simulink model "DOF4_model"  (R2023a)
settings: Solver=VariableStepAuto  StartTime=0.0  StopTime=10.0  RelTol=1e-3
values from neighbouring files (symbols this model uses):
  a = 1.8    [DOF_4_parameters.m]    (also in formulacar_params.mat; longitudinal_coefficients.m; roadcar_params.mat = 1.1)
  b = 1.7    [DOF_4_parameters.m]    (also in formulacar_params.mat; longitudinal_coefficients.m; roadcar_params.mat)
  c_damperF = 1580    [DOF_4_parameters.m]
  c_damperR = 1650    [DOF_4_parameters.m]
  F0F = m_s * (b / L) * g    (= 3740.41285714)    [DOF_4_parameters.m]
  F0R = m_s * (a / L) * g    (= 3960.43714286)    [DOF_4_parameters.m]
  g = 9.81    [DOF_4_parameters.m]    (also in formulacar_params.mat; longitudinal_coefficients.m; quarter_car_model_parameters.m; roadcar_params.mat)
  I = 1350    [DOF_4_parameters.m]    (also in formulacar_params.mat = 1500; roadcar_params.mat = 3500)
  k_springF = 37000    [DOF_4_parameters.m]
  k_springR = 47000    [DOF_4_parameters.m]
  k_tyreF = 400000    [DOF_4_parameters.m]
  k_tyreR = k_tyreF    (= 400000)    [DOF_4_parameters.m]
  m_s = 785    [DOF_4_parameters.m]    (also in quarter_car_model_parameters.m = 400)
  m_usF = 30    [DOF_4_parameters.m]
  m_usR = 35    [DOF_4_parameters.m]
  z0_tyreF = (m_s*b/L + m_usF) * g / k_tyreF    (= 0.0100867821429)    [DOF_4_parameters.m]
  z0_tyreR = (m_s*a/L + m_usF) * g / k_tyreR    (= 0.0106368428571)    [DOF_4_parameters.m]
  z_r_type = 1    [quarter_car_model_parameters.m]
libraries: simulink x1
settings Model: Creator=Cassio de Freitas  LastModifiedBy=Cassio de Freitas

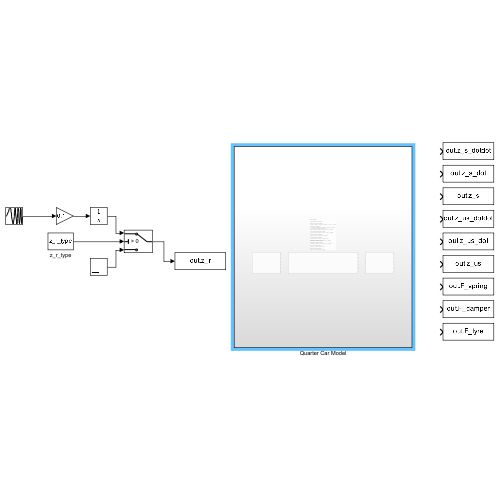
[thumbnail: Simulink's stored preview of the top-level diagram]
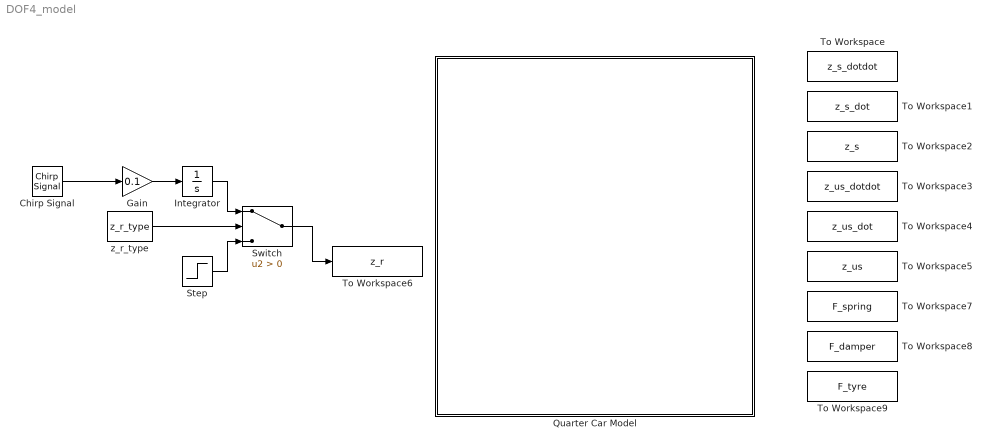
== system DOF4_model ==
  Chirp Signal : simulink/Sources/Chirp Signal  f1=0.1  T=100  f2=50
  Gain : Gain  Gain=0.1
  Integrator : Integrator
  Quarter Car Model : Subsystem
  Step : Step  After=0.1  SampleTime=1e-3
  Switch : Switch  Criteria=u2 > Threshold  SaturateOnIntegerOverflow=off  InputSameDT=off
  To Workspace : ToWorkspace  VariableName=z_s_dotdot  SaveFormat=Timeseries  SampleTime=-1
  To Workspace1 : ToWorkspace  VariableName=z_s_dot  SaveFormat=Timeseries  SampleTime=-1
  To Workspace2 : ToWorkspace  VariableName=z_s  SaveFormat=Timeseries  SampleTime=-1
  To Workspace3 : ToWorkspace  VariableName=z_us_dotdot  SaveFormat=Timeseries  SampleTime=-1
  To Workspace4 : ToWorkspace  VariableName=z_us_dot  SaveFormat=Timeseries  SampleTime=-1
  To Workspace5 : ToWorkspace  VariableName=z_us  SaveFormat=Timeseries  SampleTime=-1
  To Workspace6 : ToWorkspace  VariableName=z_r  SaveFormat=Timeseries  SampleTime=-1
  To Workspace7 : ToWorkspace  VariableName=F_spring  SaveFormat=Timeseries  SampleTime=-1
  To Workspace8 : ToWorkspace  VariableName=F_damper  SaveFormat=Timeseries  SampleTime=-1
  To Workspace9 : ToWorkspace  VariableName=F_tyre  SaveFormat=Timeseries  SampleTime=-1
  z_r_type : Constant  Value=z_r_type
  wires:
  Integrator/1 -> Switch/1
  Gain/1 -> Integrator/1
  Step/1 -> Switch/3
  z_r_type/1 -> Switch/2
  Chirp Signal/1 -> Gain/1
  Switch/1 -> To Workspace6/1

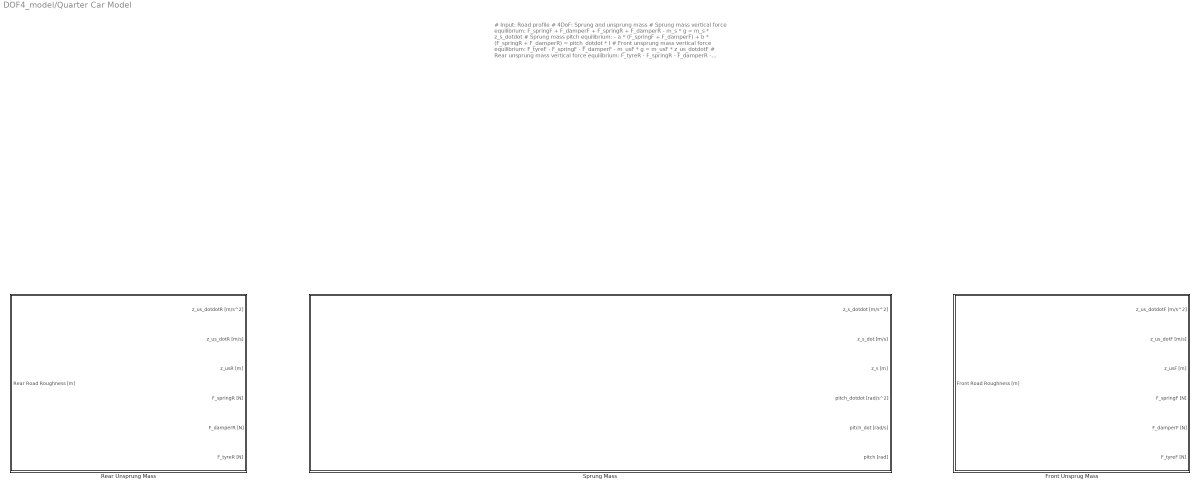
== system DOF4_model/Quarter Car Model ==
  note: # Input: Road profile
      |
      | # 4DoF: Sprung and unsprung mass
      |
      | # Sprung mass vertical force equilibrium:
      | F_springF + F_damperF + F_springR + F_damperR - m_s * g = m_s * z_s_dotdot
      |
      | # Sprung mass pitch equilibrium:
      | - a * (F_springF + F_damperF) + b * (F_springR + F_damperR) = pitch_dotdot * I
      |
      | # Front unsprung mass vertical force equilibrium:
      | F_tyreF - F_springF - F_damperF - m_usF * g = m_usF * z_us_dotdotF
      |
      | # Rear unsprung mass vertical force equilibrium:
      | F_tyreR - F_springR - F_damperR - m_usR * g = m_usR * z_us_dotdotR
      |
      | # Front spring vertical force equilibrium
      | F_springF = (z_usF - (z_s - pitch * a)) * k_springF + F0F
      |
      | # Rear spring vertical force equilibrium
      | F_springR = (z_usR - (z_s + pitch * b)) * k_springR + F0R
      |
      | # Front damper vertical force equilibrium
      | F_damperF = (z_us_dotF - (z_s_dot - pitch_dot * a)) * c_damperF
      |
      | # Rear damper vertical force equilibrium
      | F_damperR = (z_us_dotR - (z_s_dot + pitch_dot * a)) * c_damperR
      |
      | # Front tyre vertical force equilibrium
      | F_tyreF = (z_rF - z_usF +z0_tyreF) * k_tyreF
      |
      | # Rear tyre vertical force equilibrium
      | F_tyreR = (z_rR - z_usR +z0_tyreR) * k_tyreR
  Front Unsprug Mass : Subsystem
  Rear Unsprung Mass : Subsystem
  Sprung Mass : Subsystem

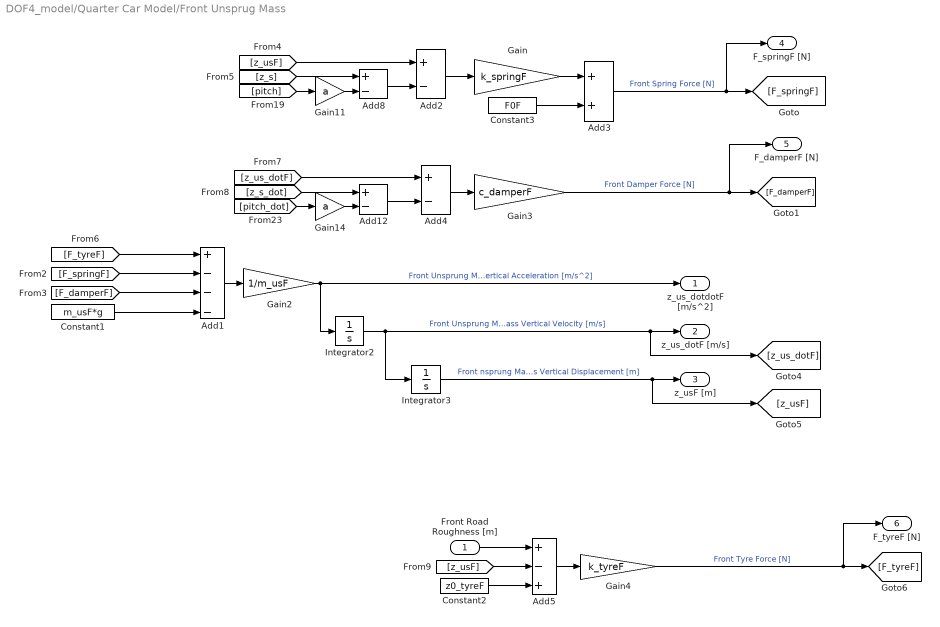
== system DOF4_model/Quarter Car Model/Front Unsprug Mass ==
  Front Road Roughness [m] : Inport
  Add1 : Sum  Inputs=+---
  Add{2,4,8,12} (4 alike) : Sum  Inputs=+-
  Add3 : Sum
  Add5 : Sum  Inputs=+-+
  Constant1 : Constant  Value=m_usF*g
  Constant2 : Constant  Value=z0_tyreF
  Constant3 : Constant  Value=F0F
  Gain : Gain  Gain=k_springF
  Gain11 : Gain  Gain=a
  Gain14 : Gain  Gain=a
  Gain2 : Gain  Gain=1/m_usF
  Gain3 : Gain  Gain=c_damperF
  Gain4 : Gain  Gain=k_tyreF
  Integrator2 : Integrator
  Integrator3 : Integrator
  z_us_dotdotF [m/s^2] : Outport
  z_us_dotF [m/s] : Outport  Port=2
  z_usF [m] : Outport  Port=3
  F_springF [N] : Outport  Port=4
  F_damperF [N] : Outport  Port=5
  F_tyreF [N] : Outport  Port=6
  wires:
  Integrator3/1 -> z_usF [m]/1, [z_usF]  "Front nsprung Mass Vertical Displacement [m]"
  Add1/1 -> Gain2/1
  [F_springF] -> Add1/2
  [F_damperF] -> Add1/3
  Integrator2/1 -> z_us_dotF [m/s]/1, [z_us_dotF], Integrator3/1  "Front Unsprung Mass Vertical Velocity [m/s]"
  Gain2/1 -> Integrator2/1, z_us_dotdotF [m/s^2]/1  "Front Unsprung Mass Vertical Acceleration [m/s^2]"
  Constant1/1 -> Add1/4
  [F_tyreF] -> Add1/1
  Gain11/1 -> Add8/2
  [z_s] -> Add8/1
  Add8/1 -> Add2/2
  Add3/1 -> F_springF [N]/1, [F_springF]  "Front Spring Force [N]"
  Gain/1 -> Add3/1
  Add4/1 -> Gain3/1
  Constant3/1 -> Add3/2
  [z_usF] -> Add2/1
  [z_us_dotF] -> Add4/1
  Gain3/1 -> F_damperF [N]/1, [F_damperF]  "Front Damper Force [N]"
  [z_s_dot] -> Add12/1
  Gain14/1 -> Add12/2
  [pitch] -> Gain11/1
  [pitch_dot] -> Gain14/1
  Add2/1 -> Gain/1
  Add12/1 -> Add4/2
  Add5/1 -> Gain4/1
  Front Road Roughness [m]/1 -> Add5/1
  [z_usF] -> Add5/2
  Constant2/1 -> Add5/3
  Gain4/1 -> F_tyreF [N]/1, [F_tyreF]  "Front Tyre Force [N]"

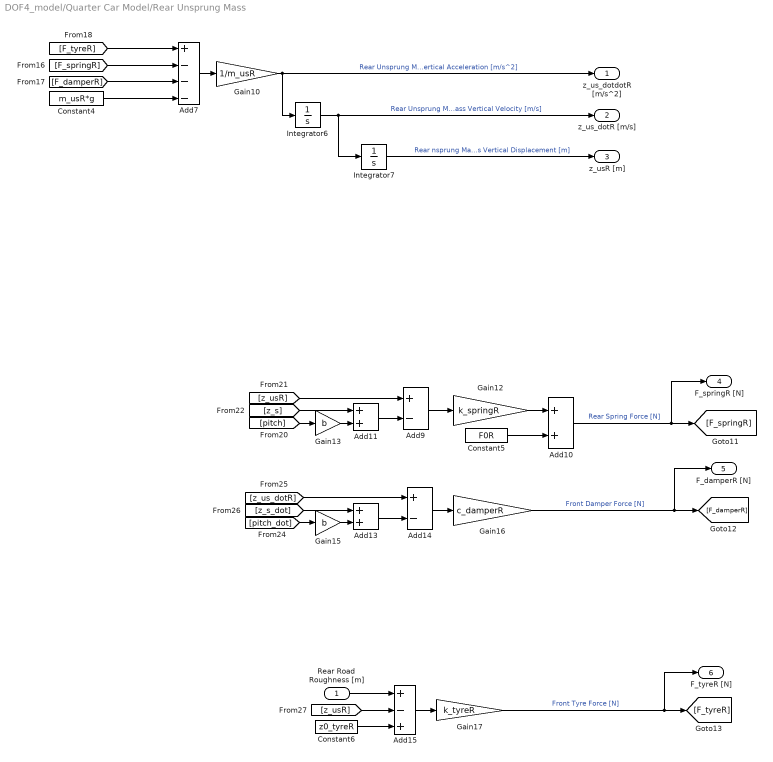
== system DOF4_model/Quarter Car Model/Rear Unsprung Mass ==
  Rear Road Roughness [m] : Inport
  Add10 : Sum
  Add11 : Sum
  Add13 : Sum
  Add14 : Sum  Inputs=+-
  Add15 : Sum  Inputs=+-+
  Add7 : Sum  Inputs=+---
  Add9 : Sum  Inputs=+-
  Constant4 : Constant  Value=m_usR*g
  Constant5 : Constant  Value=F0R
  Constant6 : Constant  Value=z0_tyreR
  Gain10 : Gain  Gain=1/m_usR
  Gain12 : Gain  Gain=k_springR
  Gain13 : Gain  Gain=b
  Gain15 : Gain  Gain=b
  Gain16 : Gain  Gain=c_damperR
  Gain17 : Gain  Gain=k_tyreR
  Integrator6 : Integrator
  Integrator7 : Integrator
  z_us_dotdotR [m/s^2] : Outport
  z_us_dotR [m/s] : Outport  Port=2
  z_usR [m] : Outport  Port=3
  F_springR [N] : Outport  Port=4
  F_damperR [N] : Outport  Port=5
  F_tyreR [N] : Outport  Port=6
  wires:
  Integrator7/1 -> z_usR [m]/1  "Rear nsprung Mass Vertical Displacement [m]"
  Add7/1 -> Gain10/1
  Gain10/1 -> Integrator6/1, z_us_dotdotR [m/s^2]/1  "Rear Unsprung Mass Vertical Acceleration [m/s^2]"
  [F_damperR] -> Add7/3
  Constant4/1 -> Add7/4
  [F_tyreR] -> Add7/1
  [F_springR] -> Add7/2
  Integrator6/1 -> z_us_dotR [m/s]/1, Integrator7/1  "Rear Unsprung Mass Vertical Velocity [m/s]"
  Add11/1 -> Add9/2
  [pitch] -> Gain13/1
  [z_s] -> Add11/1
  [z_us_dotR] -> Add14/1
  [z_s_dot] -> Add13/1
  Add9/1 -> Gain12/1
  Gain16/1 -> [F_damperR], F_damperR [N]/1  "Front Damper Force [N]"
  Add13/1 -> Add14/2
  Gain13/1 -> Add11/2
  Gain12/1 -> Add10/1
  Add14/1 -> Gain16/1
  Add10/1 -> [F_springR], F_springR [N]/1  "Rear Spring Force [N]"
  [z_usR] -> Add9/1
  Gain15/1 -> Add13/2
  Constant5/1 -> Add10/2
  [pitch_dot] -> Gain15/1
  [z_usR] -> Add15/2
  Constant6/1 -> Add15/3
  Rear Road Roughness [m]/1 -> Add15/1
  Gain17/1 -> [F_tyreR], F_tyreR [N]/1  "Front Tyre Force [N]"
  Add15/1 -> Gain17/1

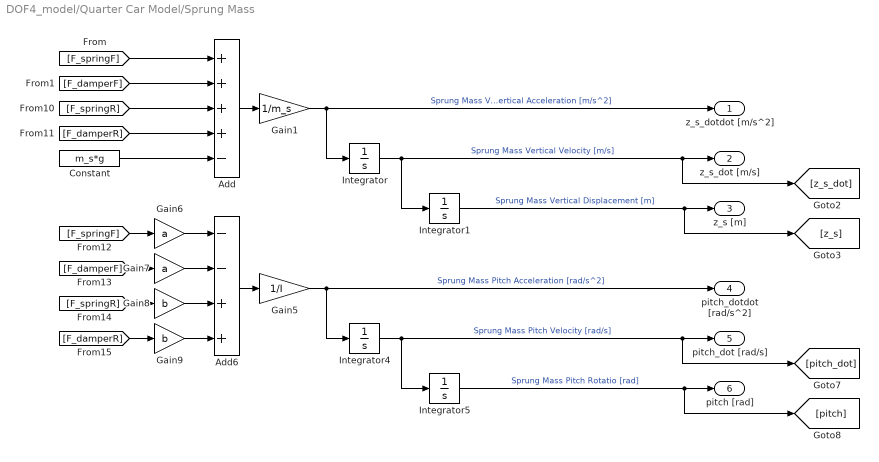
== system DOF4_model/Quarter Car Model/Sprung Mass ==
  Add : Sum  Inputs=++++-
  Add6 : Sum  Inputs=--++
  Constant : Constant  Value=m_s*g
  Gain1 : Gain  Gain=1/m_s
  Gain5 : Gain  Gain=1/I
  Gain6 : Gain  Gain=a
  Gain7 : Gain  Gain=a
  Gain8 : Gain  Gain=b
  Gain9 : Gain  Gain=b
  Integrator{,1,4..5} (4 alike) : Integrator
  z_s_dotdot [m/s^2] : Outport
  z_s_dot [m/s] : Outport  Port=2
  z_s [m] : Outport  Port=3
  pitch_dotdot [rad/s^2] : Outport  Port=4
  pitch_dot [rad/s] : Outport  Port=5
  pitch [rad] : Outport  Port=6
  wires:
  Integrator4/1 -> pitch_dot [rad/s]/1, [pitch_dot], Integrator5/1  "Sprung Mass Pitch Velocity [rad/s]"
  Gain5/1 -> pitch_dotdot [rad/s^2]/1, Integrator4/1  "Sprung Mass Pitch Acceleration [rad/s^2]"
  [F_damperR] -> Gain9/1
  [F_springR] -> Add/3
  Gain9/1 -> Add6/4
  Gain1/1 -> Integrator/1, z_s_dotdot [m/s^2]/1  "Sprung Mass Vertical Acceleration [m/s^2]"
  [F_springF] -> Add/1
  Integrator1/1 -> [z_s], z_s [m]/1  "Sprung Mass Vertical Displacement [m]"
  [F_damperF] -> Add/2
  Add/1 -> Gain1/1
  [F_damperR] -> Add/4
  Gain8/1 -> Add6/3
  Add6/1 -> Gain5/1
  Constant/1 -> Add/5
  Gain7/1 -> Add6/2
  [F_springF] -> Gain6/1
  [F_springR] -> Gain8/1
  [F_damperF] -> Gain7/1
  Gain6/1 -> Add6/1
  Integrator5/1 -> pitch [rad]/1, [pitch]  "Sprung Mass Pitch Rotatio [rad]"
  Integrator/1 -> Integrator1/1, [z_s_dot], z_s_dot [m/s]/1  "Sprung Mass Vertical Velocity [m/s]"
